simulink model "sf_msg_forwarding"  (R2017b)
settings: Solver=FixedStepDiscrete  StartTime=0.0  StopTime=10.0  FixedStep=1  RelTol=1e-3  EnableMultiTasking=on
settings Model: Creator=The MathWorks, Inc.  LastModifiedBy=The MathWorks, Inc.
settings DataIOCC: LimitDataPoints=on  SaveFormat=Array
settings OptimizationCC: LifeSpan=inf
settings DebuggingCC: SolverPrmCheckMsg=warning  AllowSymbolicDim=off  SFUnexpectedBacktrackingDiag=warning  SFNoUnconditionalDefaultTransitionDiag=warning  SFExecutionAtInitializationDiag=none
settings HardwareCC: ProdBitPerPointer=32  ProdBitPerSizeT=32  ProdBitPerPtrDiffT=32  ProdLargestAtomicFloat=None  ProdIntDivRoundTo=Undefined  ProdEndianess=Unspecified  ProdWordSize=32  ProdHWDeviceType=32-bit Generic
settings ModelReferenceCC: PropagateSignalLabelsOutOfModel=off
settings CodeAppCC: StateflowObjectComments=on
settings GRTTargetCC: TargetLangStandard=C89/C90 (ANSI)  GeneratePreprocessorConditionals=Disable all
settings ConfigComp: CovMetricSettings=dw  CovHtmlReporting=on  CovSaveCumulativeToWorkspaceVar=on  CovSaveSingleToWorkspaceVar=on  CovExternalEMLEnable=off  CovSFcnEnable=off

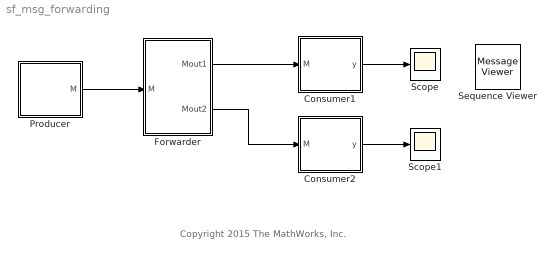
== system sf_msg_forwarding ==
  note: Copyright 2015 The MathWorks, Inc.
  Consumer1 : Stateflow chart  TreatAsAtomicUnit=on
  Consumer2 : Stateflow chart  TreatAsAtomicUnit=on
  Forwarder : Stateflow chart  TreatAsAtomicUnit=on
  Producer : Stateflow chart  TreatAsAtomicUnit=on
  Scope : Scope
  Scope1 : Scope
  Sequence Viewer : MessageViewer
  wires:
  Consumer2/1(y) -> Scope1/1
  Consumer1/1(y) -> Scope/1
  Forwarder/1(Mout1) -> Consumer1/1(M)
  Forwarder/2(Mout2) -> Consumer2/1(M)
  Producer/1(M) -> Forwarder/1(M)

== stateflow chart sf_msg_forwarding/Forwarder ==
  (default) -> (junction 6)
  (junction 6) -> (junction 5) [order 1] : M[mod(M.data,2) == 0]
  (junction 6) -> (junction 7) [order 2] : {
      | Mout2.data = M.data;
      | send(Mout2);
      | }
  (junction 5) -> (junction 4) : {
      | M.data = M.data + 3;
      | forward(M, Mout1);
      | }
  (junction 4) -> (junction 7)
  (junction 7) -> (junction 3)
  data: M input; Mout1 output; Mout2 output

== stateflow chart sf_msg_forwarding/Consumer1 ==
  state A
    on M:
    y = M.data;
  data: M input; y output

== stateflow chart sf_msg_forwarding/Producer ==
  state A
    en:
    x = 0;
    en, du:
    M.data = x;
    send(M);
    x = x + 1;
  data: M output; x local

== stateflow chart sf_msg_forwarding/Consumer2 ==
  state A
    on M:
    y = M.data;
  data: M input; y output
